simulink model "compid"  (Simulink 4.00)
settings: Solver=ode45  StartTime=0.0  StopTime=150  MaxStep=0.1  RelTol=1e-3
libraries: simulink3 x1
settings Model: LastModifiedBy=Gui

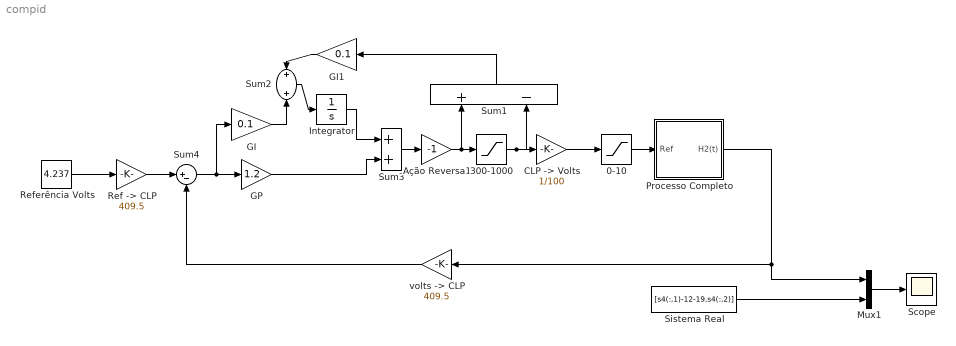
== system compid ==
  0-10 : Saturate  UpperLimit=10  LowerLimit=0  LinearizeAsGain=on
  300-1000 : Saturate  UpperLimit=1000  LowerLimit=300  LinearizeAsGain=on
  Ação Reversa1 : Gain  Gain=-1  Multiplication=Element-wise(K.*u)  SaturateOnIntegerOverflow=on
  "CLP -> Volts" : Gain  Gain=1/100  Multiplication=Element-wise(K.*u)  SaturateOnIntegerOverflow=on
  GI : Gain  Gain=0.1  Multiplication=Element-wise(K.*u)  SaturateOnIntegerOverflow=on
  GI1 : Gain  Orientation=left  Gain=0.1  Multiplication=Element-wise(K.*u)  SaturateOnIntegerOverflow=on
  GP : Gain  Gain=1.2  Multiplication=Element-wise(K.*u)  SaturateOnIntegerOverflow=on
  Integrator : Integrator  ExternalReset=none  InitialConditionSource=internal  InitialCondition=0  LimitOutput=off  UpperSaturationLimit=inf  LowerSaturationLimit=-inf  ShowSaturationPort=off  ShowStatePort=off  AbsoluteTolerance=auto
  Mux1 : Mux  Inputs=2
  Processo Completo : Subsystem
      settings: RTWFcnNameOpts=Auto  RTWFileNameOpts=Auto
  "Ref -> CLP" : Gain  Gain=409.5  Multiplication=Element-wise(K.*u)  SaturateOnIntegerOverflow=on
  Referência Volts : Constant  Value=4.237
  Scope : Scope
      settings: TimeRange=auto  YMin=-5  YMax=5  SaveToWorkspace=off  SaveName=ScopeData2  MaxDataPoints=5000
  Sistema Real : FromWorkspace  VariableName=[s4(:,1)-12-19,s4(:,2)]  SampleTime=0  OutputAfterFinalValue=Extrapolation
  Sum1 : Sum  Orientation=up  Inputs=+-  SaturateOnIntegerOverflow=on
  Sum2 : Sum  Inputs=++  SaturateOnIntegerOverflow=on
  Sum3 : Sum  Inputs=++  SaturateOnIntegerOverflow=on
  Sum4 : Sum  Inputs=|+-  SaturateOnIntegerOverflow=on
  "volts -> CLP" : Gain  Orientation=left  Gain=409.5  Multiplication=Element-wise(K.*u)  SaturateOnIntegerOverflow=on
  wires:
  GP/1 -> Sum3/2
  Sum4/1 -> GP/1, GI/1
  0-10/1 -> Processo Completo/1(Ref)
  Mux1/1 -> Scope/1
  "Ref -> CLP"/1 -> Sum4/1
  "volts -> CLP"/1 -> Sum4/2
  Referência Volts/1 -> "Ref -> CLP"/1
  Sum3/1 -> Ação Reversa1/1
  Ação Reversa1/1 -> 300-1000/1, Sum1/1
  300-1000/1 -> "CLP -> Volts"/1, Sum1/2
  "CLP -> Volts"/1 -> 0-10/1
  GI/1 -> Sum2/2
  GI1/1 -> Sum2/1
  Sum2/1 -> Integrator/1
  Integrator/1 -> Sum3/1
  Sum1/1 -> GI1/1
  Processo Completo/1("H2(t) ") -> "volts -> CLP"/1, Mux1/1
  Sistema Real/1 -> Mux1/2

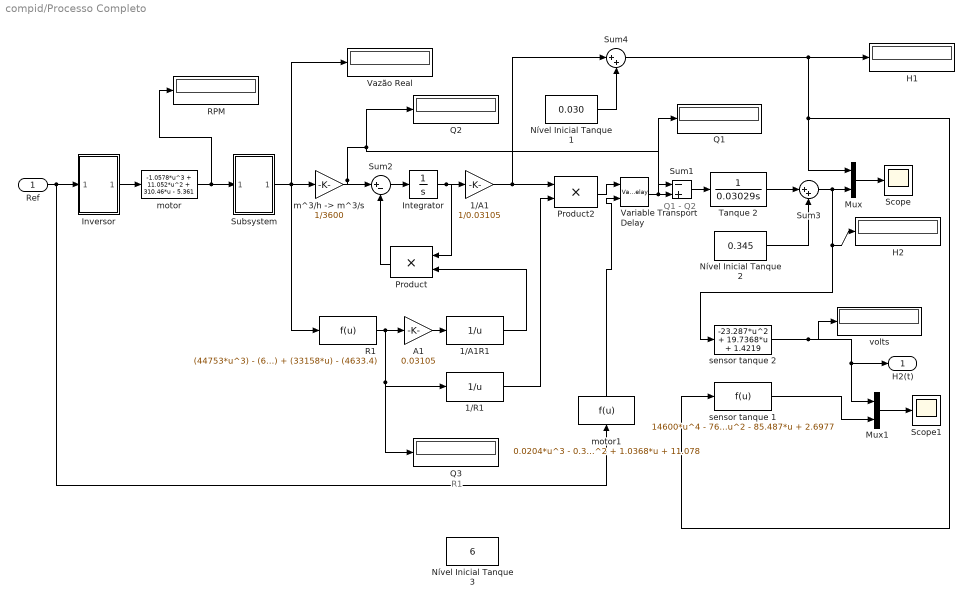
== system compid/Processo Completo ==
  note: Q1 - Q2
  note: R1
  Ref : Inport  Port=1  LatchInput=off
  1/A1 : Gain  Gain=1/0.03105  Multiplication=Element-wise(K.*u)  SaturateOnIntegerOverflow=on
  1/A1R1 : Fcn  Expr=1/u
  1/R1 : Fcn  Expr=1/u
  A1 : Gain  Gain=0.03105  Multiplication=Element-wise(K.*u)  SaturateOnIntegerOverflow=on
  H1 : Display
      settings: Format=short
  H2 : Display
      settings: Format=short
  Integrator : Integrator  ExternalReset=none  InitialConditionSource=internal  InitialCondition=0  LimitOutput=off  UpperSaturationLimit=inf  LowerSaturationLimit=-inf  ShowSaturationPort=off  ShowStatePort=off  AbsoluteTolerance=auto
  Inversor : Subsystem
      settings: RTWFcnNameOpts=Auto  RTWFileNameOpts=Auto
  Mux : Mux  Inputs=2
  Mux1 : Mux  Inputs=2
  Nível Inicial Tanque 1 : Constant  Value=0.030
  Nível Inicial Tanque 2 : Constant  Value=0.345
  Nível Inicial Tanque 3 : Constant  Value=6
  Product : Product  Orientation=left  Inputs=2  Multiplication=Element-wise(.*)  SaturateOnIntegerOverflow=on
  Product2 : Product  Inputs=2  Multiplication=Element-wise(.*)  SaturateOnIntegerOverflow=on
  Q1 : Display
      settings: Format=short
  Q2 : Display
      settings: Format=short
  Q3 : Display
      settings: Format=short
  R1 : Fcn  Expr=(44753*u^3) - (67476*u^2) + (33158*u) - (4633.4)
  RPM : Display
      settings: Format=short
  Scope : Scope
      settings: TimeRange=auto  YMin=0.161  YMax=0.1715  SaveToWorkspace=off  SaveName=ScopeData  MaxDataPoints=5000
  Scope1 : Scope
      settings: TimeRange=auto  YMin=2.4  YMax=4  SaveToWorkspace=off  MaxDataPoints=5000
  Subsystem : Subsystem
      settings: RTWFcnNameOpts=Auto  RTWFileNameOpts=Auto
  Sum1 : Sum  Inputs=-+  SaturateOnIntegerOverflow=on
  Sum2 : Sum  Inputs=|+-  SaturateOnIntegerOverflow=on
  Sum3 : Sum  Inputs=|++  SaturateOnIntegerOverflow=on
  Sum4 : Sum  Inputs=|++  SaturateOnIntegerOverflow=on
  Tanque 2 : TransferFcn  Numerator=[1]  Denominator=[0.03029 0]  AbsoluteTolerance=auto  Realization=auto
  Variable Transport Delay : VariableTransportDelay  MaximumDelay=10  InitialInput=0  MaximumPoints=1024  PadeOrder=0
  Vazão Real : Display
      settings: Format=short
  "m^3/h -> m^3/s" : Gain  Gain=1/3600  Multiplication=Element-wise(K.*u)  SaturateOnIntegerOverflow=on
  motor : Fcn  Expr=-1.0578*u^3 + 11.052*u^2 + 310.46*u - 5.361
  motor1 : Fcn  Orientation=up  Expr=0.0204*u^3 - 0.3476*u^2 + 1.0368*u + 11.078
  sensor tanque 1 : Fcn  Expr=14600*u^4 - 7625.2*u^3 + 1369.1*u^2 - 85.487*u + 2.6977
  "sensor tanque 2 " : Fcn  Expr=-23.287*u^2 + 19.7368*u + 1.4219
  "volts " : Display
      settings: Format=short
  "H2(t) " : Outport  Port=1
  wires:
  Subsystem/1(Out1) -> "m^3/h -> m^3/s"/1, Vazão Real/1, R1/1
  "m^3/h -> m^3/s"/1 -> Sum2/1, Q2/1, Sum1/1
  Integrator/1 -> Product/1, 1/A1/1
  Product/1 -> Sum2/2
  A1/1 -> 1/A1R1/1
  1/A1R1/1 -> Product/2
  R1/1 -> A1/1, 1/R1/1, Q3/1
  Sum1/1 -> Tanque 2/1
  Mux/1 -> Scope/1
  Tanque 2/1 -> Sum3/1
  Nível Inicial Tanque 2/1 -> Sum3/2
  Sum3/1 -> Mux/2, H2/1, "sensor tanque 2 "/1
  Inversor/1(Out1) -> motor/1
  Ref/1 -> motor1/1, Inversor/1(In1)
  motor/1 -> Subsystem/1(In1), RPM/1
  Mux1/1 -> Scope1/1
  Sum2/1 -> Integrator/1
  Product2/1 -> Variable Transport Delay/1
  Variable Transport Delay/1 -> Sum1/2, Q1/1
  "sensor tanque 2 "/1 -> "volts "/1, Mux1/1, "H2(t) "/1
  1/R1/1 -> Product2/2
  sensor tanque 1/1 -> Mux1/2
  1/A1/1 -> Sum4/1, Product2/1
  Sum4/1 -> H1/1, Mux/1, sensor tanque 1/1
  Nível Inicial Tanque 1/1 -> Sum4/2
  ? -> ?
  motor1/1 -> Variable Transport Delay/2

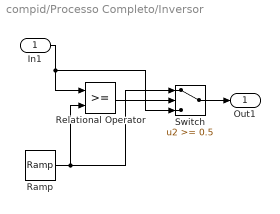
== system compid/Processo Completo/Inversor ==
  In1 : Inport  Port=1  LatchInput=off
  Ramp : simulink3/Sources/Ramp  slope=20  start=0.5  X0=0
  Relational Operator : RelationalOperator  Operator=>=
  Switch : Switch  Threshold=0.5
  Out1 : Outport  Port=1
  wires:
  In1/1 -> Relational Operator/1, Switch/3
  Ramp/1 -> Relational Operator/2, Switch/1
  Relational Operator/1 -> Switch/2
  Switch/1 -> Out1/1

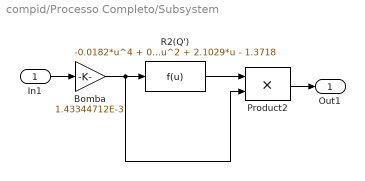
== system compid/Processo Completo/Subsystem ==
  In1 : Inport  Port=1  LatchInput=off
  Bomba : Gain  Gain=1.43344712E-3  Multiplication=Element-wise(K.*u)  SaturateOnIntegerOverflow=on
  Product2 : Product  Inputs=2  Multiplication=Element-wise(.*)  SaturateOnIntegerOverflow=on
  R2(Q') : Fcn  Expr=-0.0182*u^4 + 0.2322*u^3 - 1.0682*u^2 + 2.1029*u - 1.3718
  Out1 : Outport  Port=1
  wires:
  Bomba/1 -> R2(Q')/1, Product2/2
  R2(Q')/1 -> Product2/1
  In1/1 -> Bomba/1
  Product2/1 -> Out1/1
